simulink model "EGRVlv_DD"  (R2016b)
settings: configuration reference "CodeGenConfigSet" (kept outside this file)
values from neighbouring files (symbols this model uses):
  EGRVlv_facBattCorFacFlt_C = Calibration.Parameter    [init_EGRVlv_DD.m]    (also in init_EGRVlv_DD_SIL.m = Simulink.Parameter)
  EGRVlv_facCorStrt_C = Calibration.Parameter    [init_EGRVlv_DD.m]    (also in init_EGRVlv_DD_SIL.m = Simulink.Parameter)
  EGRVlv_rCnvHb_MAP = Calibration.Parameter    [init_EGRVlv_DD.m]    (also in init_EGRVlv_DD_SIL.m = Simulink.Parameter)
  EGRVlv_rCnvHb_MAPX = Calibration.Parameter    [init_EGRVlv_DD.m]    (also in init_EGRVlv_DD_SIL.m = Simulink.Parameter)
  EGRVlv_rCnvHb_MAPY = Calibration.Parameter    [init_EGRVlv_DD.m]    (also in init_EGRVlv_DD_SIL.m = Simulink.Parameter)
  EGRVlv_rCnvPsNrmHb_CUR = Calibration.Parameter    [init_EGRVlv_DD.m]    (also in init_EGRVlv_DD_SIL.m = Simulink.Parameter)
  EGRVlv_rCnvPsNrmHb_CURX = Calibration.Parameter    [init_EGRVlv_DD.m]    (also in init_EGRVlv_DD_SIL.m = Simulink.Parameter)
  EGRVlv_rCnvPsNrmPWM_CUR = Calibration.Parameter    [init_EGRVlv_DD.m]    (also in init_EGRVlv_DD_SIL.m = Simulink.Parameter)
  EGRVlv_rCnvPsNrmPWM_CURX = Calibration.Parameter    [init_EGRVlv_DD.m]    (also in init_EGRVlv_DD_SIL.m = Simulink.Parameter)
  EGRVlv_rCnvPWM_MAP = Calibration.Parameter    [init_EGRVlv_DD.m]    (also in init_EGRVlv_DD_SIL.m = Simulink.Parameter)
  EGRVlv_rCnvPWM_MAPX = Calibration.Parameter    [init_EGRVlv_DD.m]    (also in init_EGRVlv_DD_SIL.m = Simulink.Parameter)
  EGRVlv_rCnvPWM_MAPY = Calibration.Parameter    [init_EGRVlv_DD.m]    (also in init_EGRVlv_DD_SIL.m = Simulink.Parameter)
  EGRVlv_rPwmOutMax_C = Calibration.Parameter    [init_EGRVlv_DD.m]    (also in init_EGRVlv_DD_SIL.m = Simulink.Parameter)
  EGRVlv_rPwmOutMin_C = Calibration.Parameter    [init_EGRVlv_DD.m]    (also in init_EGRVlv_DD_SIL.m = Simulink.Parameter)
  EGRVlv_stPwrStgDiaDis_C = Calibration.Parameter    [init_EGRVlv_DD.m]    (also in init_EGRVlv_DD_SIL.m = Simulink.Parameter)
  EGRVlv_stPwrStgDis_C = Calibration.Parameter    [init_EGRVlv_DD.m]    (also in init_EGRVlv_DD_SIL.m = Simulink.Parameter)
  EGRVlv_swtHwSel_C = Calibration.Parameter    [init_EGRVlv_DD.m]    (also in init_EGRVlv_DD_SIL.m = Simulink.Parameter)
  EGRVlv_swtPwmOutBattCor_C = Calibration.Parameter    [init_EGRVlv_DD.m]    (also in init_EGRVlv_DD_SIL.m = Simulink.Parameter)
  EGRVlv_tiPs_C = Calibration.Parameter    [init_EGRVlv_DD.m]    (also in init_EGRVlv_DD_SIL.m = Simulink.Parameter)
undefined symbols (not defined in the file or in its folder): EngState_conv
libraries: CXLib x6
settings Model: Creator=lvzhanghui  LastModifiedBy=zhulinfeng
settings ConfigSetRef: SourceLocation=Base Workspace

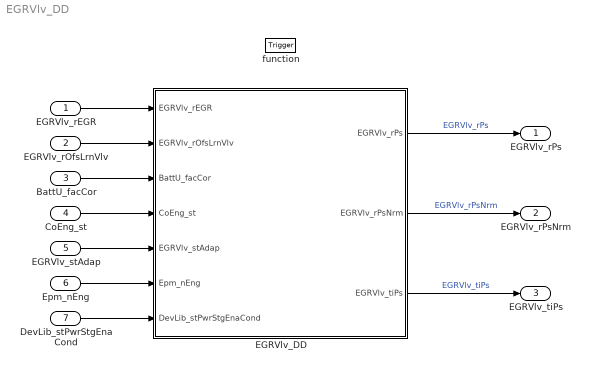
== system EGRVlv_DD ==
  EGRVlv_rEGR : Inport  Tag=%  Description=Control value for the EGR valve  OutMin=-100  OutMax=100  OutDataTypeStr=Prc_100_rate
  EGRVlv_rOfsLrnVlv : Inport  Tag=%  Description=Control value for offset learning  Port=2  OutMin=-100  OutMax=100  OutDataTypeStr=Prc_100_rate
  BattU_facCor : Inport  Description=Battery correction factor  Port=3  OutMin=-32  OutMax=31.9  OutDataTypeStr=Factor
  CoEng_st : Inport  Description=Engine coordinator state  Port=4  OutDataTypeStr=Enum: EngState_conv
  EGRVlv_stAdap : Inport  Description=Status of offset learning  Port=5  OutMin=0  OutMax=65535  OutDataTypeStr=State_uint16
  Epm_nEng : Inport  Tag=rpm  Description=Engine speed  Port=6  OutMin=0  OutMax=6000  OutDataTypeStr=EngSpeed_rpm
  DevLib_stPwrStgEnaCond : Inport  Description=Control unit status relevant to power stage deactivation/error diagnosis  Port=7  OutMin=0  OutMax=65535  OutDataTypeStr=State_uint16
  function : TriggerPort  TriggerType=function-call  VariantControl=Variant
  EGRVlv_DD : Subsystem
  EGRVlv_rPs : Outport  Tag=%  Description=Duty cycle to power stage  OutMin=-100  OutMax=100  OutDataTypeStr=Prc_100_rate
  EGRVlv_rPsNrm : Outport  Tag=%  Description=Normalized value of EGRVLv_rPSNrm  Port=2  OutMin=-100  OutMax=100  OutDataTypeStr=Prc_100_rate
  EGRVlv_tiPs : Outport  Tag=us  Description=signal period duration  Port=3  OutMin=-107374182  OutMax=107374182  OutDataTypeStr=Time_PwmHigh_us
  wires:
  EGRVlv_rEGR/1 -> EGRVlv_DD/1(EGRVlv_rEGR)
  EGRVlv_rOfsLrnVlv/1 -> EGRVlv_DD/2(EGRVlv_rOfsLrnVlv)
  BattU_facCor/1 -> EGRVlv_DD/3(BattU_facCor)
  CoEng_st/1 -> EGRVlv_DD/4(CoEng_st)
  EGRVlv_stAdap/1 -> EGRVlv_DD/5(EGRVlv_stAdap)
  Epm_nEng/1 -> EGRVlv_DD/6(Epm_nEng)
  DevLib_stPwrStgEnaCond/1 -> EGRVlv_DD/7(DevLib_stPwrStgEnaCond)
  EGRVlv_DD/1(EGRVlv_rPs) -> EGRVlv_rPs/1  "EGRVlv_rPs"
  EGRVlv_DD/2(EGRVlv_rPsNrm) -> EGRVlv_rPsNrm/1  "EGRVlv_rPsNrm"
  EGRVlv_DD/3(EGRVlv_tiPs) -> EGRVlv_tiPs/1  "EGRVlv_tiPs"

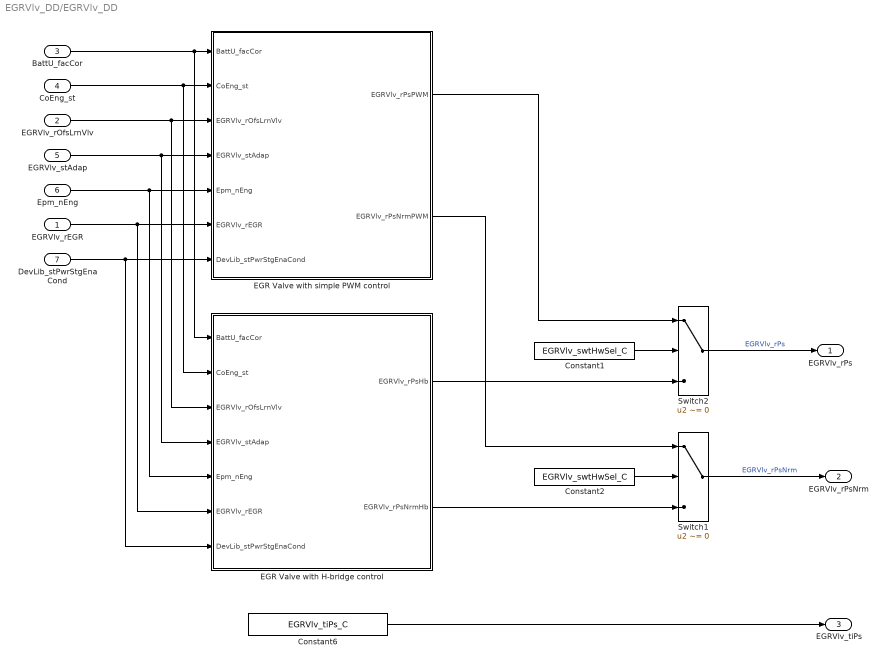
== system EGRVlv_DD/EGRVlv_DD ==
  EGRVlv_rEGR : Inport  Tag=%
  EGRVlv_rOfsLrnVlv : Inport  Tag=%  Port=2
  BattU_facCor : Inport  Tag=%  Port=3
  CoEng_st : Inport  Tag=%  Port=4
  EGRVlv_stAdap : Inport  Port=5
  Epm_nEng : Inport  Tag=%  Port=6
  DevLib_stPwrStgEnaCond : Inport  Tag=%  Port=7
  Constant1 : Constant  Value=EGRVlv_swtHwSel_C  SampleTime=-1
  Constant2 : Constant  Value=EGRVlv_swtHwSel_C  SampleTime=-1
  Constant6 : Constant  Value=EGRVlv_tiPs_C  SampleTime=-1
  EGR Valve with H-bridge control : Subsystem
  EGR Valve with simple PWM control : Subsystem
  Switch1 : Switch  Criteria=u2 ~= 0
  Switch2 : Switch  Criteria=u2 ~= 0
  EGRVlv_rPs : Outport  Tag=kPa
  EGRVlv_rPsNrm : Outport  Tag=kPa  Port=2
  EGRVlv_tiPs : Outport  Tag=%  Port=3
  wires:
  EGR Valve with simple PWM control/1(EGRVlv_rPsPWM) -> Switch2/1
  Epm_nEng/1 -> EGR Valve with H-bridge control/5(Epm_nEng), EGR Valve with simple PWM control/5(Epm_nEng)
  Constant1/1 -> Switch2/2
  EGR Valve with H-bridge control/2(EGRVlv_rPsNrmHb) -> Switch1/3
  EGRVlv_rOfsLrnVlv/1 -> EGR Valve with H-bridge control/3(EGRVlv_rOfsLrnVlv), EGR Valve with simple PWM control/3(EGRVlv_rOfsLrnVlv)
  EGR Valve with H-bridge control/1(EGRVlv_rPsHb) -> Switch2/3
  Switch1/1 -> EGRVlv_rPsNrm/1  "EGRVlv_rPsNrm"
  DevLib_stPwrStgEnaCond/1 -> EGR Valve with H-bridge control/7(DevLib_stPwrStgEnaCond), EGR Valve with simple PWM control/7(DevLib_stPwrStgEnaCond)
  EGRVlv_stAdap/1 -> EGR Valve with H-bridge control/4(EGRVlv_stAdap), EGR Valve with simple PWM control/4(EGRVlv_stAdap)
  EGR Valve with simple PWM control/2(EGRVlv_rPsNrmPWM) -> Switch1/1
  BattU_facCor/1 -> EGR Valve with H-bridge control/1(BattU_facCor), EGR Valve with simple PWM control/1(BattU_facCor)
  EGRVlv_rEGR/1 -> EGR Valve with H-bridge control/6(EGRVlv_rEGR), EGR Valve with simple PWM control/6(EGRVlv_rEGR)
  Constant2/1 -> Switch1/2
  Switch2/1 -> EGRVlv_rPs/1  "EGRVlv_rPs"
  CoEng_st/1 -> EGR Valve with H-bridge control/2(CoEng_st), EGR Valve with simple PWM control/2(CoEng_st)
  Constant6/1 -> EGRVlv_tiPs/1

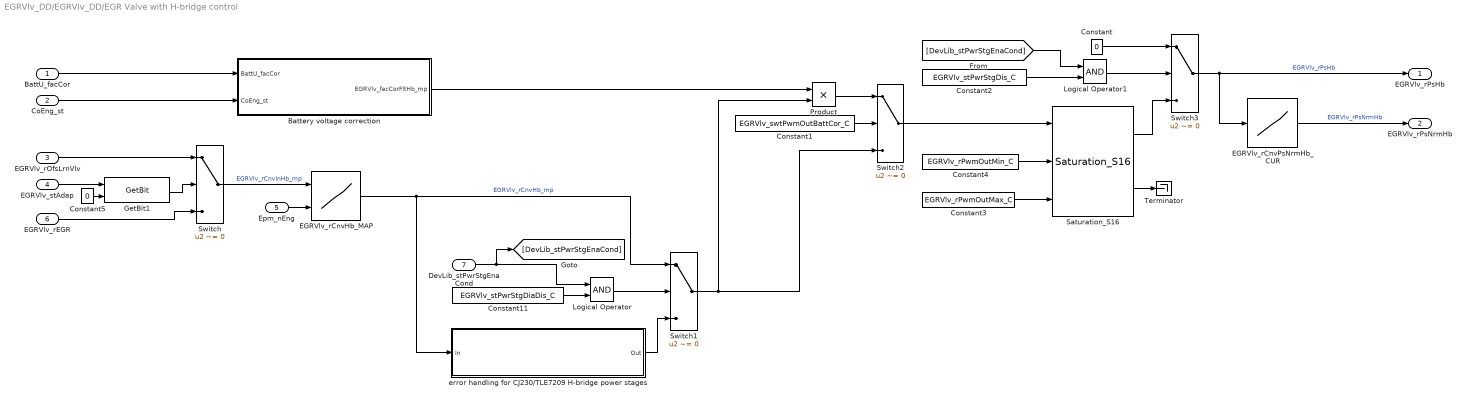
== system EGRVlv_DD/EGRVlv_DD/EGR Valve with H-bridge control ==
  BattU_facCor : Inport  Tag=%
  CoEng_st : Inport  Tag=%  Port=2
  EGRVlv_rOfsLrnVlv : Inport  Tag=%  Port=3
  EGRVlv_stAdap : Inport  Port=4
  Epm_nEng : Inport  Tag=%  Port=5
  EGRVlv_rEGR : Inport  Tag=%  Port=6
  DevLib_stPwrStgEnaCond : Inport  Tag=%  Port=7
  Battery voltage correction : Subsystem
  Constant : Constant  Value=0  OutDataTypeStr=Prc_100_rate
  Constant1 : Constant  Value=EGRVlv_swtPwmOutBattCor_C  SampleTime=-1
  Constant11 : Constant  Value=EGRVlv_stPwrStgDiaDis_C  SampleTime=-1
  Constant2 : Constant  Value=EGRVlv_stPwrStgDis_C  SampleTime=-1
  Constant3 : Constant  Value=EGRVlv_rPwmOutMax_C  SampleTime=-1
  Constant4 : Constant  Value=EGRVlv_rPwmOutMin_C  SampleTime=-1
  Constant5 : Constant  Value=0  OutDataTypeStr=uint8
  EGRVlv_rCnvHb_MAP : Lookup_n-D  BreakpointsForDimension1=EGRVlv_rCnvHb_MAPX  BreakpointsForDimension2=EGRVlv_rCnvHb_MAPY  Table=EGRVlv_rCnvHb_MAP  TableDataTypeStr=Inherit: Inherit from 'Table data'  ExtrapMethod=Clip  InternalRulePriority=Speed  OutDataTypeStr=Inherit: Inherit from 'Table data'  RndMeth=Simplest  SaturateOnIntegerOverflow=on
  EGRVlv_rCnvPsNrmHb_CUR : Lookup_n-D  NumberOfTableDimensions=1  BreakpointsForDimension1=EGRVlv_rCnvPsNrmHb_CURX  Table=EGRVlv_rCnvPsNrmHb_CUR  TableDataTypeStr=Inherit: Inherit from 'Table data'  ExtrapMethod=Clip  InternalRulePriority=Speed  OutDataTypeStr=Inherit: Inherit from 'Table data'  RndMeth=Simplest  SaturateOnIntegerOverflow=on
  GetBit1 : CXLib/GetBit  dataTypeString=uint16  dataLength=0
      settings: AttributesFormatString=Get bit from %<dataTypeString>
  Logical Operator : Logic  AllPortsSameDT=off  OutDataTypeStr=boolean
  Logical Operator1 : Logic  AllPortsSameDT=off  OutDataTypeStr=boolean
  Product : Product  OutDataTypeStr=Prc_100_rate  SaturateOnIntegerOverflow=on
  Saturation_S16 : CXLib/Saturation_S16
  Switch{,1..3} (4 alike) : Switch  Criteria=u2 ~= 0
  Terminator : Terminator
  error handling for CJ230/TLE7209 H-bridge power stages : Subsystem
  EGRVlv_rPsHb : Outport  Tag=kPa
  EGRVlv_rPsNrmHb : Outport  Tag=kPa  Port=2
  wires:
  Switch/1 -> EGRVlv_rCnvHb_MAP/1  "EGRVlv_rCnvInHb_mp"
  EGRVlv_rEGR/1 -> Switch/3
  EGRVlv_rOfsLrnVlv/1 -> Switch/1
  Epm_nEng/1 -> EGRVlv_rCnvHb_MAP/2
  EGRVlv_rCnvHb_MAP/1 -> Switch1/1, error handling for CJ230/TLE7209 H-bridge power stages/1(In)  "EGRVlv_rCnvHb_mp"
  Logical Operator/1 -> Switch1/2
  Constant2/1 -> Logical Operator1/2
  [DevLib_stPwrStgEnaCond] -> Logical Operator1/1
  EGRVlv_rCnvPsNrmHb_CUR/1 -> EGRVlv_rPsNrmHb/1  "EGRVlv_rPsNrmHb"
  error handling for CJ230/TLE7209 H-bridge power stages/1(Out) -> Switch1/3
  Constant/1 -> Switch3/1
  Constant4/1 -> Saturation_S16/2
  GetBit1/1 -> Switch/2
  Switch1/1 -> Product/2, Switch2/3
  Constant1/1 -> Switch2/2
  Battery voltage correction/1(EGRVlv_facCorFltHb_mp) -> Product/1
  Constant3/1 -> Saturation_S16/3
  Logical Operator1/1 -> Switch3/2
  DevLib_stPwrStgEnaCond/1 -> [DevLib_stPwrStgEnaCond], Logical Operator/1
  Constant11/1 -> Logical Operator/2
  Product/1 -> Switch2/1
  Saturation_S16/1 -> Switch3/3
  Switch2/1 -> Saturation_S16/1
  Switch3/1 -> EGRVlv_rPsHb/1, EGRVlv_rCnvPsNrmHb_CUR/1  "EGRVlv_rPsHb"
  BattU_facCor/1 -> Battery voltage correction/1(BattU_facCor)
  CoEng_st/1 -> Battery voltage correction/2(CoEng_st)
  Saturation_S16/2 -> Terminator/1
  Constant5/1 -> GetBit1/2
  EGRVlv_stAdap/1 -> GetBit1/1

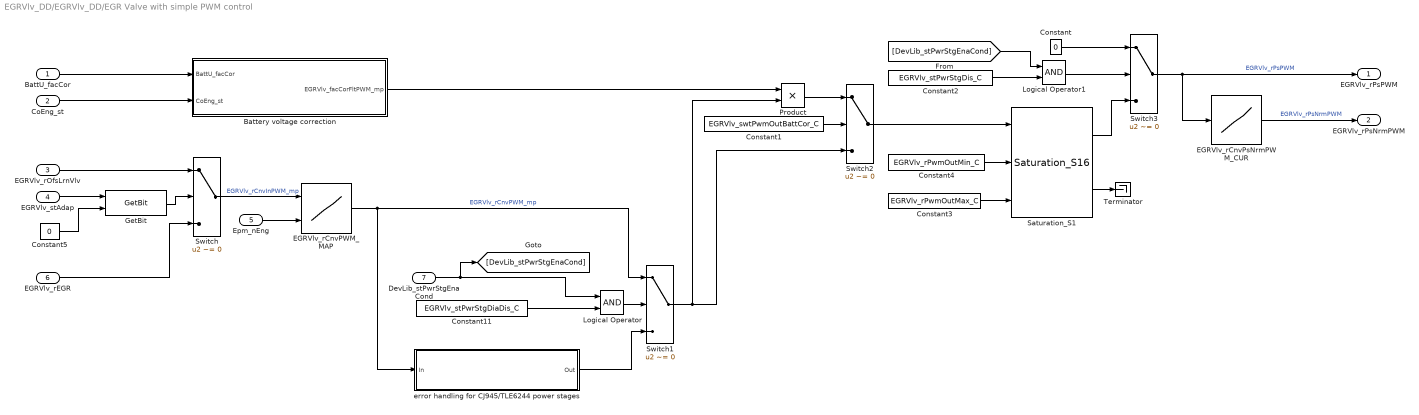
== system EGRVlv_DD/EGRVlv_DD/EGR Valve with simple PWM control ==
  BattU_facCor : Inport  Tag=%
  CoEng_st : Inport  Tag=%  Port=2
  EGRVlv_rOfsLrnVlv : Inport  Tag=%  Port=3
  EGRVlv_stAdap : Inport  Port=4
  Epm_nEng : Inport  Tag=%  Port=5
  EGRVlv_rEGR : Inport  Tag=%  Port=6
  DevLib_stPwrStgEnaCond : Inport  Tag=%  Port=7
  Battery voltage correction : Subsystem
  Constant : Constant  Value=0  OutDataTypeStr=Inherit: Inherit via back propagation
  Constant1 : Constant  Value=EGRVlv_swtPwmOutBattCor_C  SampleTime=-1
  Constant11 : Constant  Value=EGRVlv_stPwrStgDiaDis_C  SampleTime=-1
  Constant2 : Constant  Value=EGRVlv_stPwrStgDis_C  SampleTime=-1
  Constant3 : Constant  Value=EGRVlv_rPwmOutMax_C  SampleTime=-1
  Constant4 : Constant  Value=EGRVlv_rPwmOutMin_C  SampleTime=-1
  Constant5 : Constant  Value=0  OutDataTypeStr=uint8
  EGRVlv_rCnvPWM_MAP : Lookup_n-D  BreakpointsForDimension1=EGRVlv_rCnvPWM_MAPX  BreakpointsForDimension2=EGRVlv_rCnvPWM_MAPY  Table=EGRVlv_rCnvPWM_MAP  TableDataTypeStr=Inherit: Inherit from 'Table data'  ExtrapMethod=Clip  InternalRulePriority=Speed  OutDataTypeStr=Inherit: Inherit from 'Table data'  RndMeth=Simplest  SaturateOnIntegerOverflow=on
  EGRVlv_rCnvPsNrmPWM_CUR : Lookup_n-D  NumberOfTableDimensions=1  BreakpointsForDimension1=EGRVlv_rCnvPsNrmPWM_CURX  Table=EGRVlv_rCnvPsNrmPWM_CUR  TableDataTypeStr=Inherit: Inherit from 'Table data'  ExtrapMethod=Clip  InternalRulePriority=Speed  OutDataTypeStr=Inherit: Inherit from 'Table data'  RndMeth=Simplest  SaturateOnIntegerOverflow=on
  GetBit : CXLib/GetBit  dataTypeString=uint16  dataLength=0
      settings: AttributesFormatString=Get bit from %<dataTypeString>
  Logical Operator : Logic  AllPortsSameDT=off  OutDataTypeStr=boolean
  Logical Operator1 : Logic  AllPortsSameDT=off  OutDataTypeStr=boolean
  Product : Product  OutDataTypeStr=Prc_100_rate  SaturateOnIntegerOverflow=on
  Saturation_S1 : CXLib/Saturation_S16
  Switch{,1..3} (4 alike) : Switch  Criteria=u2 ~= 0
  Terminator : Terminator
  error handling for CJ945/TLE6244 power stages : Subsystem
  EGRVlv_rPsPWM : Outport  Tag=kPa
  EGRVlv_rPsNrmPWM : Outport  Tag=kPa  Port=2
  wires:
  Switch/1 -> EGRVlv_rCnvPWM_MAP/1  "EGRVlv_rCnvInPWM_mp"
  EGRVlv_rEGR/1 -> Switch/3
  EGRVlv_rOfsLrnVlv/1 -> Switch/1
  Epm_nEng/1 -> EGRVlv_rCnvPWM_MAP/2
  EGRVlv_rCnvPWM_MAP/1 -> Switch1/1, error handling for CJ945/TLE6244 power stages/1(In)  "EGRVlv_rCnvPWM_mp"
  Logical Operator/1 -> Switch1/2
  Constant2/1 -> Logical Operator1/2
  [DevLib_stPwrStgEnaCond] -> Logical Operator1/1
  EGRVlv_rCnvPsNrmPWM_CUR/1 -> EGRVlv_rPsNrmPWM/1  "EGRVlv_rPsNrmPWM"
  error handling for CJ945/TLE6244 power stages/1(Out) -> Switch1/3
  Constant/1 -> Switch3/1
  Constant4/1 -> Saturation_S1/2
  GetBit/1 -> Switch/2
  Switch1/1 -> Product/2, Switch2/3
  Constant1/1 -> Switch2/2
  Battery voltage correction/1(EGRVlv_facCorFltPWM_mp) -> Product/1
  Constant3/1 -> Saturation_S1/3
  Logical Operator1/1 -> Switch3/2
  DevLib_stPwrStgEnaCond/1 -> [DevLib_stPwrStgEnaCond], Logical Operator/1
  Constant11/1 -> Logical Operator/2
  Product/1 -> Switch2/1
  Saturation_S1/1 -> Switch3/3
  Switch2/1 -> Saturation_S1/1
  Switch3/1 -> EGRVlv_rPsPWM/1, EGRVlv_rCnvPsNrmPWM_CUR/1  "EGRVlv_rPsPWM"
  BattU_facCor/1 -> Battery voltage correction/1(BattU_facCor)
  CoEng_st/1 -> Battery voltage correction/2(CoEng_st)
  Saturation_S1/2 -> Terminator/1
  Constant5/1 -> GetBit/2
  EGRVlv_stAdap/1 -> GetBit/1

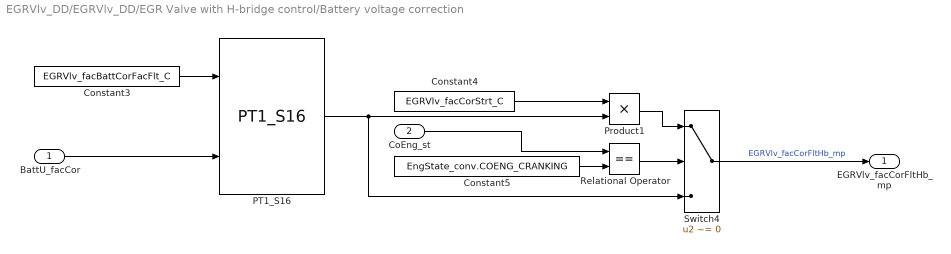
== system EGRVlv_DD/EGRVlv_DD/EGR Valve with H-bridge control/Battery voltage correction ==
  BattU_facCor : Inport  Tag=%
  CoEng_st : Inport  Tag=%  Port=2
  Constant3 : Constant  Value=EGRVlv_facBattCorFacFlt_C  SampleTime=-1
  Constant4 : Constant  Value=EGRVlv_facCorStrt_C  SampleTime=-1
  Constant5 : Constant  Value=EngState_conv.COENG_CRANKING  OutDataTypeStr=Enum:EngState_conv
  PT1_S16 : CXLib/PT1_S16
  Product1 : Product  OutDataTypeStr=Factor  SaturateOnIntegerOverflow=on
  Relational Operator : RelationalOperator  Operator===  OutDataTypeStr=boolean  RndMeth=Simplest
  Switch4 : Switch  Criteria=u2 ~= 0
  EGRVlv_facCorFltHb_mp : Outport  Tag=kPa
  wires:
  Constant3/1 -> PT1_S16/1
  Constant4/1 -> Product1/1
  Product1/1 -> Switch4/1
  PT1_S16/1 -> Product1/2, Switch4/3
  Constant5/1 -> Relational Operator/2
  CoEng_st/1 -> Relational Operator/1
  Relational Operator/1 -> Switch4/2
  Switch4/1 -> EGRVlv_facCorFltHb_mp/1  "EGRVlv_facCorFltHb_mp"
  BattU_facCor/1 -> PT1_S16/2

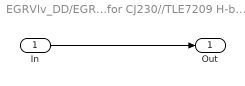
== system EGRVlv_DD/EGRVlv_DD/EGR Valve with H-bridge control/error handling for CJ230//TLE7209 H-bridge power stages ==
  In : Inport  Tag=%
  Out : Outport  Tag=kPa
  wires:
  In/1 -> Out/1

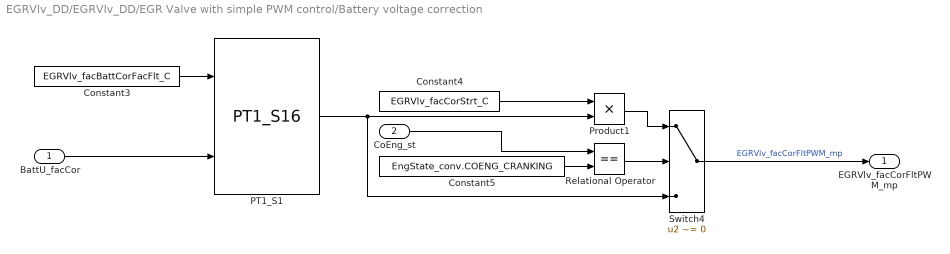
== system EGRVlv_DD/EGRVlv_DD/EGR Valve with simple PWM control/Battery voltage correction ==
  BattU_facCor : Inport  Tag=%
  CoEng_st : Inport  Tag=%  Port=2
  Constant3 : Constant  Value=EGRVlv_facBattCorFacFlt_C  SampleTime=-1
  Constant4 : Constant  Value=EGRVlv_facCorStrt_C  SampleTime=-1
  Constant5 : Constant  Value=EngState_conv.COENG_CRANKING  OutDataTypeStr=Enum:EngState_conv
  PT1_S1 : CXLib/PT1_S16
  Product1 : Product  OutDataTypeStr=Factor  SaturateOnIntegerOverflow=on
  Relational Operator : RelationalOperator  Operator===  OutDataTypeStr=boolean  RndMeth=Simplest
  Switch4 : Switch  Criteria=u2 ~= 0
  EGRVlv_facCorFltPWM_mp : Outport  Tag=kPa
  wires:
  Constant3/1 -> PT1_S1/1
  Constant4/1 -> Product1/1
  Product1/1 -> Switch4/1
  PT1_S1/1 -> Switch4/3, Product1/2
  Constant5/1 -> Relational Operator/2
  CoEng_st/1 -> Relational Operator/1
  Relational Operator/1 -> Switch4/2
  Switch4/1 -> EGRVlv_facCorFltPWM_mp/1  "EGRVlv_facCorFltPWM_mp"
  BattU_facCor/1 -> PT1_S1/2

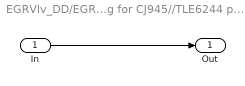
== system EGRVlv_DD/EGRVlv_DD/EGR Valve with simple PWM control/error handling for CJ945//TLE6244 power stages ==
  In : Inport  Tag=%
  Out : Outport  Tag=kPa
  wires:
  In/1 -> Out/1
